simulink model "spwm"  (R2015b)
settings: Solver=VariableStepAuto  StartTime=0.0  StopTime=0.05  RelTol=1e-3
libraries: powerlib_meascontrol x1
settings Model: Creator=u19d36  LastModifiedBy=u19d36

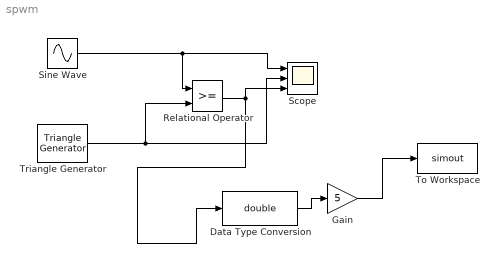
== system spwm ==
  Data Type Conversion : DataTypeConversion  OutDataTypeStr=double
  Gain : Gain  Gain=5
  Relational Operator : RelationalOperator  OutDataTypeStr=boolean
  Scope : Scope  NumInputPorts=3
  Sine Wave : Sin  SineType=Sample based  Frequency=2*pi  Samples=1000  SampleTime=1e-5
  To Workspace : ToWorkspace  VariableName=simout  SaveFormat=Timeseries  SampleTime=-1
  Triangle Generator : powerlib_meascontrol/Pulse & Signal Generators/Triangle Generator  Freq=800  Phase=90  Ts=1e-5
  wires:
  Sine Wave/1 -> Relational Operator/1, Scope/1
  Triangle Generator/1 -> Scope/2, Relational Operator/2
  Relational Operator/1 -> Data Type Conversion/1, Scope/3
  Data Type Conversion/1 -> Gain/1
  Gain/1 -> To Workspace/1
